simulink model "untitled"  (R2023b)
settings: Solver=VariableStepAuto  StartTime=0.0  StopTime=10.0  RelTol=1e-3
settings Model: Creator=IIITB  LastModifiedBy=IIITB

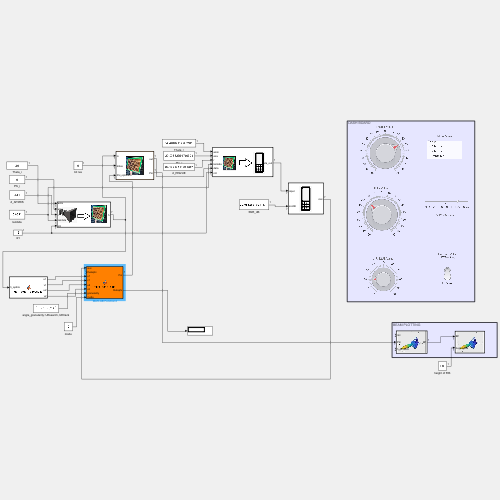
[thumbnail: Simulink's stored preview of the top-level diagram]
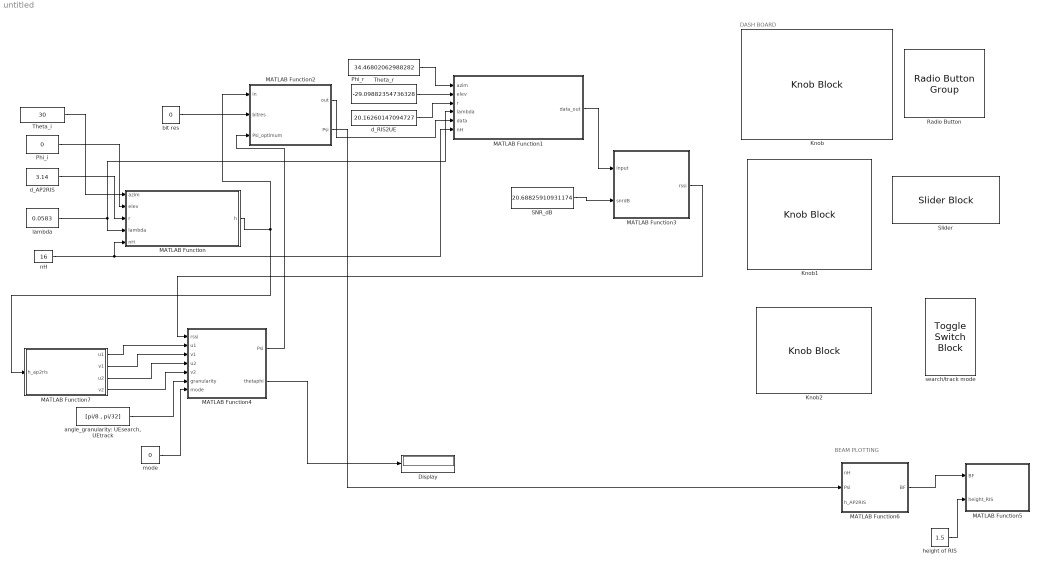
== system untitled ==
  note: BEAM PLOTTING
  note: DASH BOARD
  Display : Display
  Knob : KnobBlock  ScaleMin=-90  ScaleMax=90
  Knob1 : KnobBlock  ScaleMin=-90  ScaleMax=90
  Knob2 : KnobBlock
  MATLAB Function : MATLAB Function  TreatAsAtomicUnit=on
  MATLAB Function1 : MATLAB Function  TreatAsAtomicUnit=on
  MATLAB Function2 : MATLAB Function  TreatAsAtomicUnit=on
  MATLAB Function3 : MATLAB Function  TreatAsAtomicUnit=on
  MATLAB Function4 : MATLAB Function  TreatAsAtomicUnit=on
  MATLAB Function5 : MATLAB Function  TreatAsAtomicUnit=on
  MATLAB Function6 : MATLAB Function  TreatAsAtomicUnit=on
  MATLAB Function7 : MATLAB Function  TreatAsAtomicUnit=on
  Phi_i : Constant  Value=0  OutMin=-90  OutMax=+90
  Phi_r : Constant  Value=-29.09882354736328  OutMin=-90  OutMax=+90
  Radio Button : RadioButtonGroup  SelectedLabel=1-bit res  ButtonGroupName=Group
      settings: Values={{'1-bit res', '2-bit res', 'infinite res'}, [0 1 2]}
  SNR_dB : Constant  Value=20.68825910931174
  Slider : SliderBlock  LabelPosition=Bottom  ScaleMin=-10  ScaleMax=30
  Theta_i : Constant  Value=30  OutMin=-90  OutMax=+90
  Theta_r : Constant  Value=34.46802062988282  OutMin=-90  OutMax=+90
  "angle_granularity: UEsearch, UEtrack" : Constant  Value=[pi/8 , pi/32]
  bit res : Constant  Value=0  OutMin=1  OutMax=3
  d_AP2RIS : Constant  Value=3.14
  d_RIS2UE : Constant  Value=20.16260147094727
  height of RIS : Constant  Value=1.5
  lambda : Constant  Value=0.0583
  mode : Constant  Value=0
  nH : Constant  Value=16
  search/track mode : ToggleSwitchBlock
      settings: Values={{'UE Search', 'UE Tracking'}, [0 1]}
  wires:
  MATLAB Function/1(h) -> MATLAB Function2/1(in), MATLAB Function7/1(h_ap2ris)
  MATLAB Function1/1(data_out) -> MATLAB Function3/1(input)
  Phi_i/1 -> MATLAB Function/2(elev)
  Theta_i/1 -> MATLAB Function/1(azim)
  d_AP2RIS/1 -> MATLAB Function/3(r)
  d_RIS2UE/1 -> MATLAB Function1/3(r)
  lambda/1 -> MATLAB Function/4(lambda), MATLAB Function1/4(lambda)
  Theta_r/1 -> MATLAB Function1/1(azim)
  Phi_r/1 -> MATLAB Function1/2(elev)
  MATLAB Function2/1(out) -> MATLAB Function1/5(data)
  bit res/1 -> MATLAB Function2/2(bitres)
  SNR_dB/1 -> MATLAB Function3/2(snrdB)
  MATLAB Function6/1(BF) -> MATLAB Function5/1(BF)
  MATLAB Function2/2(Psi) -> MATLAB Function6/2(Psi)
  height of RIS/1 -> MATLAB Function5/2(height_RIS)
  nH/1 -> MATLAB Function/5(nH), MATLAB Function1/6(nH)
  MATLAB Function4/1(Psi) -> MATLAB Function2/3(Psi_optimum)
  MATLAB Function7/1(u1) -> MATLAB Function4/2(u1)
  MATLAB Function7/2(v1) -> MATLAB Function4/3(v1)
  MATLAB Function7/3(u2) -> MATLAB Function4/4(u2)
  MATLAB Function7/4(v2) -> MATLAB Function4/5(v2)
  MATLAB Function4/2(thetaphi) -> Display/1
  "angle_granularity: UEsearch, UEtrack"/1 -> MATLAB Function4/6(granularity)
  mode/1 -> MATLAB Function4/7(mode)
  MATLAB Function3/1(rssi) -> MATLAB Function4/1(rssi)

== matlab function untitled/MATLAB Function1 ==
  data: azim input; elev input; r input; lambda input; data_out output; data input; nH input
function data_out = LosChan1x256_RIS2UE(azim,elev,r,lambda,data,nH) % size(data) = [ 256x1 ] 

    arv1 = exp(-1i*pi*(0:(nH-1))*sin(azim)*cos(elev)).'; % RIS Reflector Array Phase Response
    arv2 = exp(-1i*pi*(0:(nH-1))*sin(elev)).';
    arv  = kron(arv1,arv2);
    initial_random_phase = exp(1i*2*pi*rand);
    h  = arv*initial_random_phase;
    data_out = data(:).*h(:); % size(data_out) = [256x1]
    % fspl = 4*pi*r/lambda;
    % h = h/fspl;

== matlab function untitled/MATLAB Function ==
  data: h output; azim input; elev input; r input; lambda input; nH input
function h = LosChan256x1_AP2RIS(azim,elev,r,lambda,nH)

    arv1 = exp(-1i*pi*(0:(nH-1))*sin(azim)*cos(elev)).'; % RIS Reflector Array Phase Response
    arv2 = exp(-1i*pi*(0:(nH-1))*sin(elev)).';
    arv  = kron(arv1,arv2);
    initial_random_phase = exp(1i*2*pi*rand);
    h  = arv*initial_random_phase; % size(h) = [256 x 1] 
    %fspl = 4*pi*r/lambda;
    %h = h/fspl;

== matlab function untitled/MATLAB Function2 ==
  data: in input; bitres input; Psi_optimum input; out output; Psi output
function [out,Psi] = RIS(in, bitres,Psi_optimum)

switch bitres
    case 0 % 1-bit res
        Psi_suboptimum_1bit = zeros(size(Psi_optimum)); 
        for i = 1: length(Psi_optimum)
            if(abs(Psi_optimum(i))>=pi/2 )
                Psi_suboptimum_1bit(i) = pi;
            end
        end
        Psi = Psi_suboptimum_1bit;

     case 1  % 2-bit res
        Psi_suboptimum_2bit = floor(2*(1+Psi_optimum/pi));
        Psi_suboptimum_2bit(Psi_suboptimum_2bit == 0) = -3*pi/4;
        Psi_suboptimum_2bit(Psi_suboptimum_2bit == 1) = -pi/4;
        Psi_suboptimum_2bit(Psi_suboptimum_2bit == 2) = pi/4;
        Psi_suboptimum_2bit(Psi_suboptimum_2bit == 3) = 3*pi/4; 
        Psi = Psi_suboptimum_2bit;

     case 2  % infinite-bit res(optimum)
        Psi = Psi_optimum;
end
out = in.*exp(1i.*Psi);

== matlab function untitled/MATLAB Function3 ==
  data: input input; rssi output; snrdB input
function rssi  = UE(input,snrdB)
    snr = 10^(snrdB/10);
    rx = sum(input);
    noise = (1/sqrt(2))*(randn(size(input)) + 1i*randn(size(input)));
    rxN = sqrt(snr/2)*(rx) + noise;
    rssi = abs(rxN).^2;

== matlab function untitled/MATLAB Function4 ==
  data: Psi output; rssi input; u1 input; v1 input; u2 input; v2 input; thetaphi output; granularity input; mode input
function [Psi,thetaphi]  = psi_updating_algo(rssi,u1,v1,u2,v2, granularity,mode)
% size(u1) = [256x1]
% size(u2) = [256x1]
% size(v1) = [1x2]
% size(v2) = [1x2]
% size(thetaphi) = [2x1]
% granularity = [ueSearchGranularity, ueTrackGranularity];
% mode = 0 => UE Search mode , mode = 1 => UE Track mode 

    gran = granularity(mode+1);
    if(mode == 0)
        theta_sweep= gran/2:gran:pi/2-gran/2;
        phi_sweep= gran/2:gran:pi/2-gran/2;
        for i = 1: length(theta_sweep)
            for j = 1: length(phi_sweep)
                Psi = u1*v1*[theta_sweep(i);phi_sweep(j)] + u2*v2*[theta_sweep(i);phi_sweep(j)]; % Converting [theta,phi] to Psi
                pause(0.1);
                rssi_coarse(i,j)= rssi;
            end
        end
        [~,maxidx]= max(rssi_coarse(:));
        coarse_theta = mod(maxidx,length(theta_sweep));
        coarse_phi = floor(maxidx/length(theta_sweep));
        mode = 1;
    else
        theta_sweep = coarse_theta -gran/2: coarse_theta +gran/2;
        phi_sweep = coarse_phi -gran/2: coarse_phi +gran/2;
        for i = 1: length(theta_sweep)
            for j = 1: length(phi_sweep)
                Psi = u1*v1*[theta_sweep(i);phi_sweep(j)] + u2*v2*[theta_sweep(i);phi_sweep(j)]; % Converting [theta,phi] to Psi
                pause(0.1);
                rssi_coarse(i,j)= rssi;
            end
        end
        [~,maxidx]= max(rssi_coarse(:));
        theta = mod(maxidx,length(theta_sweep));
        phi = floor(maxidx/length(theta_sweep));
        mode = 1;

    end

== matlab function untitled/MATLAB Function5 ==
  data: BF input; height_RIS input
function plot_BF_pattern(BF,height_RIS)

    global azimGrid; 
    global elevGrid; 
    norm_BF = BF/max(max(BF));
    magnification_factor = 4;
    [X, Y, Z]   = sph2cart(-azimGrid,-elevGrid, magnification_factor*norm_BF);
    colormap turbo
    BFsurface = surf(X,Y,Z+height_RIS, norm_BF);

    view([1 1 1])
    set(BFsurface,'LineStyle','none','FaceAlpha',0.5,'Tag','3D polar plot');

== matlab function untitled/MATLAB Function6 ==
  data: nH input; BF output; Psi input; h_AP2RIS input
function BF = BF_pattern(nH,Psi,h_AP2RIS)

    global angleGrid;
    global azimGrid; 
    global elevGrid; 
    global gradations; %#ok<*GVMIS>

    angleGrid= linspace(-pi/2,pi/2,gradations);
    [azimGrid,elevGrid] = meshgrid(angleGrid, angleGrid);
    BF = zeros(size(azimGrid));


    h_subopt = conj(h_AP2RIS).*exp(-1i*Psi);

    for i = 1:length(angleGrid)
        for j = 1:length(angleGrid)

            arrayResponseVector1 = exp(-1i*pi*(0:(nH-1))*sin(azimGrid(i,j))*cos(elevGrid(i,j))).';
            arrayResponseVector2 = exp(-1i*pi*(0:(nH-1))*sin(elevGrid(i,j))).';
            arrayResponseVector = kron(arrayResponseVector1,arrayResponseVector2);
            BF(i,j) = abs(sum(arrayResponseVector.* h_subopt )); % Taking the dot product
        end
        % disp([num2str(i) ' out of ' num2str(length(angleGrid)) ]);
    end
    BF =BF./(nH*nH);
    BF = BF.^2;

== matlab function untitled/MATLAB Function7 ==
  data: h_ap2ris input; u1 output; v1 output; u2 output; v2 output
function [u1,v1,u2,v2] = gen_eigen_directions(h_ap2ris)

[u,s,v] = svd(A);
u1 = u(1,:);
u2 = u(:,2);
v1 = v(:,1);
v2 = v(:,2);
